simulink model "Voltage_Control_Induction_Motor"  (R2025a)
settings: Solver=ode23tb  StartTime=0.0  StopTime=10.0  MaxStep=1e-4  RelTol=1e-3
libraries: spsControlledVoltageSourceLib x3, simulink x2, spsAsynchronousMachineSIUnitsLib x1, sps_lib x1
settings Model: Creator=Jawad  LastModifiedBy=Jawad

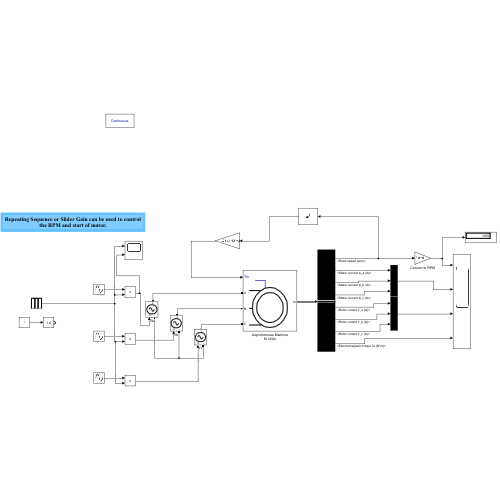
[thumbnail: Simulink's stored preview of the top-level diagram]
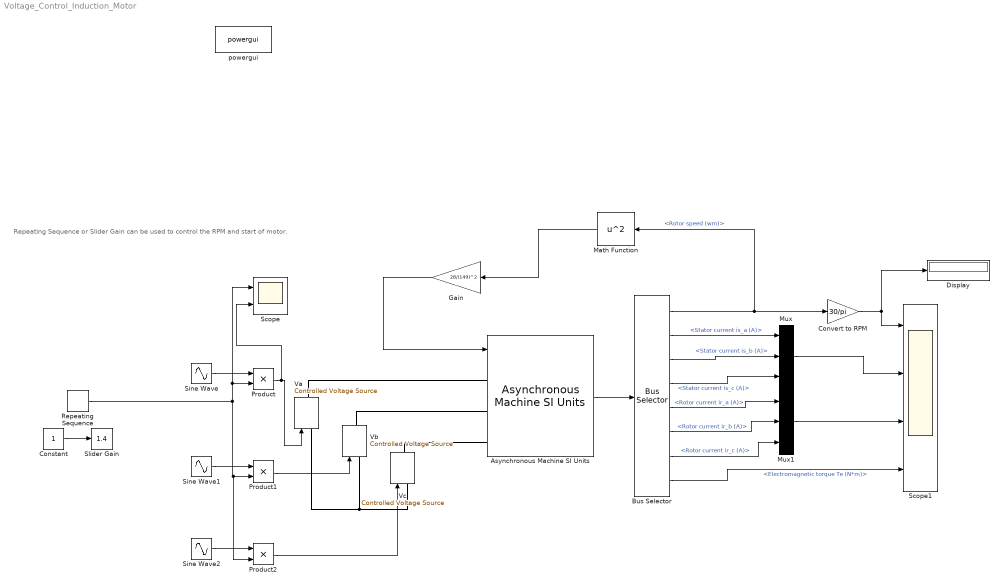
== system Voltage_Control_Induction_Motor ==
  note: Repeating Sequence or Slider Gain can be used to control the RPM and start of motor.
  Asynchronous Machine SI Units : spsAsynchronousMachineSIUnitsLib/Asynchronous Machine SI Units  RotorType=Squirrel-cage  PresetModel="15:  5.4 HP (4KW)   400 V  50Hz 1430 RPM"  MechanicalLoad=Torque Tm  ShowDetailedParameters=on  ReferenceFrame=Rotor  Units=SI  MeasurementBus=off  NominalParameters=[4000 400 50]  VoltageRatio=1  Stator=[1.405 0.005839]  Rotor=[1.395 0.005839]  Cage1=[0.4155 0.002066]  Cage2=[0.4168 0.0003495]  Lm=0.1722  Mechanical=[0.0131 0.002985 2]  PolePairs=2  InitialConditions=[1 0 0 0 0 0 0 0]  SimulateSaturation=off  Saturation=[14.03593122, 27.81365428, 53.79336849, 72.68890987, 97.98006896, 148.6815601, 215.7428561, 302.9841135, 428.7778367 ; 230, 322, 414, 460, 506, 552, 598, 644, 690]  LoadFlowParameters=1492000  TsPowergui=0  TsBlock=-1  IterativeModel=Trapezoidal non iterative  IterativeDiscreteModel=Trapezoidal non iterative  Pmec=1.492e+006
  Bus Selector : BusSelector  OutputSignals=Mechanical.Rotor speed (wm),Stator measurements.Stator current is_a (A),Stator measurements.Stator current is_b (A),Stator measurements.Stator current is_c (A),Rotor measurements.Rotor current ir_a (A),Rotor measurements.Rotor current ir_b (A),Rotor measurements.Rotor current ir_c (A),Mechanical.Electromagnetic torque Te (N*m)
  Constant : Constant
  Convert to RPM : Gain  Gain=30/pi
  Display : Display
  Gain : Gain  Gain=28/(149)^2
  Math Function : Math  Operator=square
  Mux : Mux  Inputs=3
  Mux1 : Mux  Inputs=3
  Product : Product
  Product1 : Product
  Product2 : Product
  Repeating Sequence : simulink/Sources/Repeating Sequence  rep_seq_t=[0 0.2 10]  rep_seq_y=[0 1 1]
  Scope : Scope  NumInputPorts=2
      settings: ActiveDisplayYMinimum=-0.12499999999999997  ActiveDisplayYMaximum=1.125
  Scope1 : Scope  NumInputPorts=4
      settings: ActiveDisplayString=4  Title=Electromagnetic Torque  ActiveDisplayYMinimum=-5.2353561703917819  ActiveDisplayYMaximum=47.118205533526044
  Sine Wave : Sin  Amplitude=327  Frequency=50*2*pi  SampleTime=0
  Sine Wave1 : Sin  Amplitude=327  Frequency=50*2*pi  Phase=-120*(pi/180)  SampleTime=0
  Sine Wave2 : Sin  Amplitude=327  Frequency=50*2*pi  Phase=120*(pi/180)  SampleTime=0
  Slider Gain : simulink/Math Operations/Slider Gain  gain=1.4  low=0  high=2
  Va : spsControlledVoltageSourceLib/Controlled Voltage Source  Initialize=on  Source_Type=AC  Amplitude=0  Phase=0  Frequency=0  Measurements=None
  Vb : spsControlledVoltageSourceLib/Controlled Voltage Source  Initialize=on  Source_Type=AC  Amplitude=0  Phase=0  Frequency=0  Measurements=None
  Vc : spsControlledVoltageSourceLib/Controlled Voltage Source  Initialize=on  Source_Type=AC  Amplitude=0  Phase=0  Frequency=0  Measurements=None
  powergui : sps_lib/powergui  Priority=1  SimulationMode=Continuous  SampleTime=50e-6  frequency=60  Iterations=50  frequencyindice=50  Pbase=100e6  ErrMax=1e-4  UnitsV=kV  UnitsW=MW  buscounter=0  FunctionMessages=off  echomessages=off  EnableUseOfTLC=off  CurrentSourceSwitches=off  DisableSnubberDevices=off  DisableRonSwitches=off  DisableVfSwitches=off  DisplayEquations=off  AutomaticDiscreteSolvers=off  SolverType=Tustin/Backward Euler (TBE)  Interpol=off  ExternalGateDelay=off  methode=off  Ts=100  x0status=blocks  SPID=on  SwTol=0  HookPort=off  NonlinearTolerance=1e-4  nMaxIteration=100  ContinueOnMaxIteration=off  RestoreLinks=warning  ResistiveCurrentMeasurement=off  Frange=[0:2:500]  Ylog=off  Xlog=on  ShowGrid=off  save=off  variable=ZData  structure=0  ZoomFFT=off  StartTime=0.0  cycles=1  DisplayStyle=1  fundamental=60  FreqAxis=off  MaxFrequency=1000  frequencyindicesteady=1  RmsSteady=1  display=off
  wires:
  Bus Selector/5 -> Mux1/1  "<Rotor current ir_a (A)>"
  Asynchronous Machine SI Units/1 -> Bus Selector/1
  Convert to RPM/1 -> Scope1/1, Display/1
  Mux1/1 -> Scope1/3
  Bus Selector/1 -> Math Function/1, Convert to RPM/1  "<Rotor speed (wm)>"
  Bus Selector/6 -> Mux1/2  "<Rotor current ir_b (A)>"
  Gain/1 -> Asynchronous Machine SI Units/1
  Bus Selector/2 -> Mux/1  "<Stator current is_a (A)>"
  Math Function/1 -> Gain/1
  Mux/1 -> Scope1/2
  Bus Selector/3 -> Mux/2  "<Stator current is_b (A)>"
  Bus Selector/7 -> Mux1/3  "<Rotor current ir_c (A)>"
  Bus Selector/4 -> Mux/3  "<Stator current is_c (A)>"
  Bus Selector/8 -> Scope1/4  "<Electromagnetic torque Te (N*m)>"
  Sine Wave/1 -> Product/1
  Product/1 -> Scope/2, Va/1
  Sine Wave1/1 -> Product1/1
  Sine Wave2/1 -> Product2/1
  Product1/1 -> Vb/1
  Product2/1 -> Vc/1
  Constant/1 -> Slider Gain/1
  Repeating Sequence/1 -> Product2/2, Product1/2, Scope/1, Product/2
  connections:
  Vc/RConn1 -- Asynchronous Machine SI Units/LConn3
  Vb/RConn1 -- Asynchronous Machine SI Units/LConn2
  Va/RConn1 -- Asynchronous Machine SI Units/LConn1
  Vc/LConn1 -- Vb/LConn1 -- Va/LConn1
